simulink model "L2_Step1"  (R2021b)
settings: Solver=FixedStepDiscrete  StartTime=0.0  StopTime=inf  FixedStep=0.01  RelTol=1e-3
model workspace (MATLAB code in the model file):
  | IgnitionOff = 0;
  | IgnitionACC = 1;
  | IgnitionOnEngineOn = 2;
  | KeyAbsent = 5;
  | 
  | Active = 1;
  | Not_Active = 0;
settings Model: Creator=Ekrem Fidan  LastModifiedBy=Ekrem Fidan

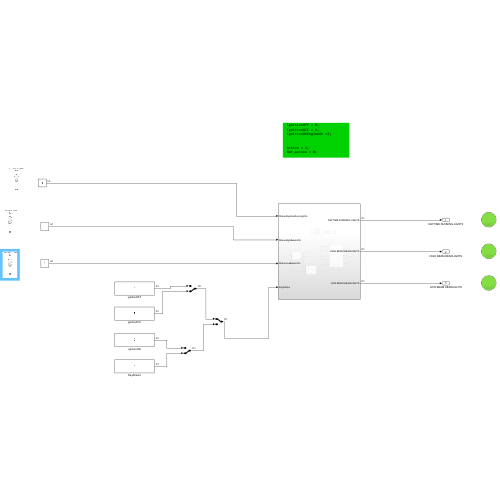
[thumbnail: Simulink's stored preview of the top-level diagram]
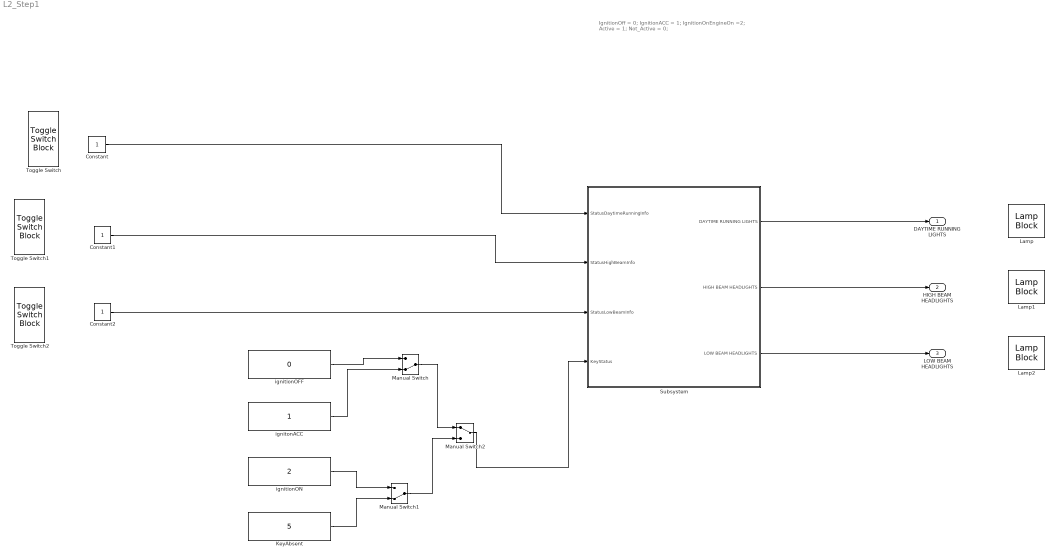
== system L2_Step1 ==
  note: IgnitionOff = 0;
      | IgnitionACC = 1;
      | IgnitionOnEngineOn =2;
      |
      | Active = 1;
      | Not_Active = 0;
  Constant : Constant
  Constant1 : Constant
  Constant2 : Constant
  KeyAbsent : Constant  Value=5  SampleTime=-1
  Lamp : LampBlock  LabelPosition=Hide
  Lamp1 : LampBlock  LabelPosition=Hide
  Lamp2 : LampBlock  LabelPosition=Hide
  Manual Switch : ManualSwitch  CurrentSetting=0
  Manual Switch1 : ManualSwitch  CurrentSetting=0
  Manual Switch2 : ManualSwitch
  Subsystem : Subsystem
  Toggle Switch : ToggleSwitchBlock
      settings: Values={{'Off', 'On'}, [0 1]}
  Toggle Switch1 : ToggleSwitchBlock
      settings: Values={{'Off', 'On'}, [0 1]}
  Toggle Switch2 : ToggleSwitchBlock
      settings: Values={{'Off', 'On'}, [0 1]}
  ignitionOFF : Constant  Value=0  SampleTime=-1
  ignitionON : Constant  Value=2  SampleTime=-1
  ignitonACC : Constant  SampleTime=-1
  DAYTIME RUNNING LIGHTS : Outport
  HIGH BEAM HEADLIGHTS : Outport  Port=2
  LOW BEAM HEADLIGHTS : Outport  Port=3
  wires:
  ignitionOFF/1 -> Manual Switch/1
  ignitonACC/1 -> Manual Switch/2
  ignitionON/1 -> Manual Switch1/1
  KeyAbsent/1 -> Manual Switch1/2
  Manual Switch/1 -> Manual Switch2/1
  Manual Switch1/1 -> Manual Switch2/2
  Constant/1 -> Subsystem/1(StatusDaytimeRunningInfo)
  Constant1/1 -> Subsystem/2(StatusHighBeamInfo)
  Constant2/1 -> Subsystem/3(StatusLowBeamInfo)
  Manual Switch2/1 -> Subsystem/4(KeyStatus)
  Subsystem/1(DAYTIME RUNNING LIGHTS) -> DAYTIME RUNNING LIGHTS/1
  Subsystem/2(HIGH BEAM HEADLIGHTS) -> HIGH BEAM HEADLIGHTS/1
  Subsystem/3(LOW BEAM HEADLIGHTS) -> LOW BEAM HEADLIGHTS/1

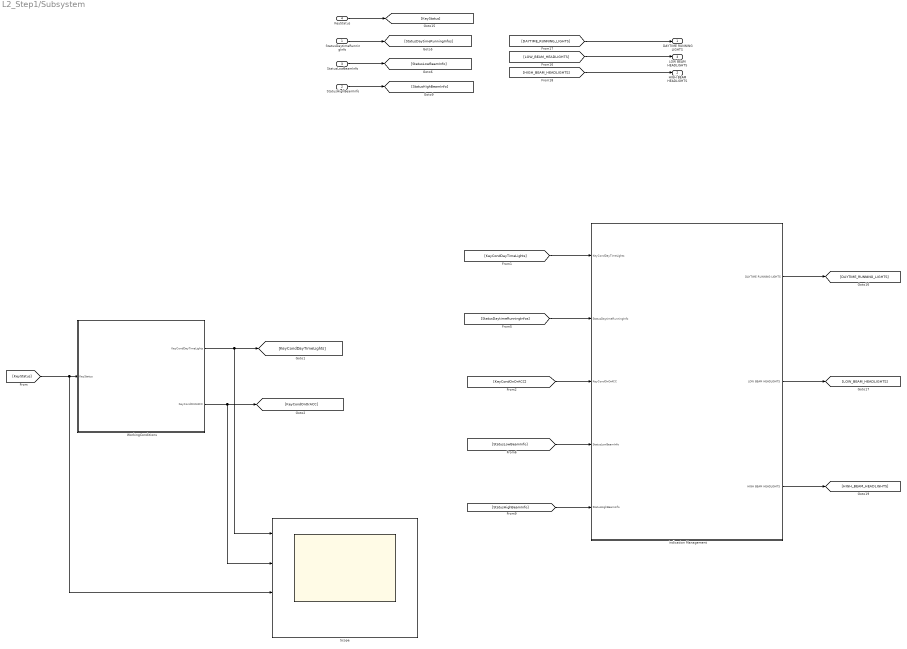
== system L2_Step1/Subsystem ==
  StatusDaytimeRunningInfo : Inport
  StatusHighBeamInfo : Inport  Port=2
  StatusLowBeamInfo : Inport  Port=3
  KeyStatus : Inport  Port=4
  Scope : Scope  NumInputPorts=4
  WorkingConditions : Subsystem
  indication Management : Subsystem
  DAYTIME RUNNING LIGHTS : Outport
  HIGH BEAM HEADLIGHTS : Outport  Port=2
  LOW BEAM HEADLIGHTS : Outport  Port=3
  wires:
  [HIGH_BEAM_HEADLIGHTS] -> HIGH BEAM HEADLIGHTS/1
  WorkingConditions/2(KeyCondOnOrACC) -> Scope/2, [KeyCondOnOrACC]
  [StatusHighBeamInfo] -> indication Management/5(StatusHighBeamInfo)
  [KeyCondOnOrACC] -> indication Management/3(KeyCondOnOrACC)
  indication Management/2(LOW BEAM HEADLIGHTS) -> [LOW_BEAM_HEADLIGHTS]
  WorkingConditions/1(KeyCondDayTimeLights) -> Scope/1, [KeyCondDayTimeLights]
  [DAYTIME_RUNNING_LIGHTS] -> DAYTIME RUNNING LIGHTS/1
  [StatusLowBeamInfo] -> indication Management/4(StatusLowBeamInfo)
  StatusDaytimeRunningInfo/1 -> [StatusDaytimeRunningInfos]
  indication Management/1(DAYTIME RUNNING LIGHTS) -> [DAYTIME_RUNNING_LIGHTS]
  [KeyCondDayTimeLights] -> indication Management/1(KeyCondDayTimeLights)
  [StatusDaytimeRunningInfos] -> indication Management/2(StatusDaytimeRunningInfo)
  StatusLowBeamInfo/1 -> [StatusLowBeamInfo]
  indication Management/3(HIGH BEAM HEADLIGHTS) -> [HIGH_BEAM_HEADLIGHTS]
  StatusHighBeamInfo/1 -> [StatusHighBeamInfo]
  [LOW_BEAM_HEADLIGHTS] -> LOW BEAM HEADLIGHTS/1
  KeyStatus/1 -> [KeyStatus]
  [KeyStatus] -> Scope/3, WorkingConditions/1(KeyStatus)

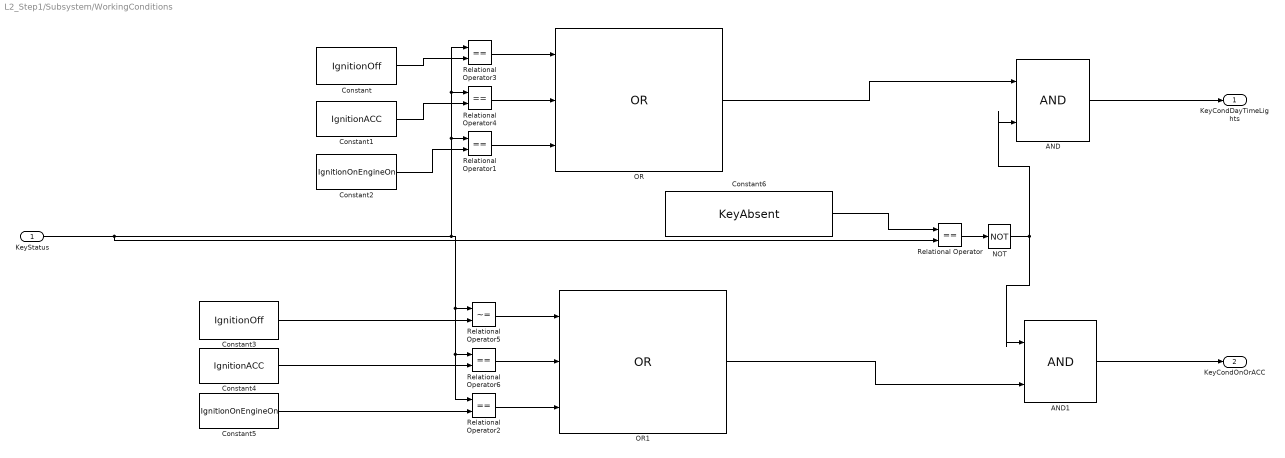
== system L2_Step1/Subsystem/WorkingConditions ==
  KeyStatus : Inport
  AND : Logic  IconShape=distinctive  AllPortsSameDT=off  OutDataTypeStr=boolean
  AND1 : Logic  IconShape=distinctive  AllPortsSameDT=off  OutDataTypeStr=boolean
  Constant : Constant  Value=IgnitionOff  SampleTime=-1
  Constant1 : Constant  Value=IgnitionACC  SampleTime=-1
  Constant2 : Constant  Value=IgnitionOnEngineOn  SampleTime=-1
  Constant3 : Constant  Value=IgnitionOff  SampleTime=-1
  Constant4 : Constant  Value=IgnitionACC  SampleTime=-1
  Constant5 : Constant  Value=IgnitionOnEngineOn  SampleTime=-1
  Constant6 : Constant  Value=KeyAbsent
  NOT : Logic  Operator=NOT  IconShape=distinctive  AllPortsSameDT=off  OutDataTypeStr=boolean
  OR : Logic  Operator=OR  Inputs=3  IconShape=distinctive  AllPortsSameDT=off  OutDataTypeStr=boolean
  OR1 : Logic  Operator=OR  Inputs=3  IconShape=distinctive  AllPortsSameDT=off  OutDataTypeStr=boolean
  Relational Operator{,1..4,6} (6 alike) : RelationalOperator  Operator===  OutDataTypeStr=boolean  RndMeth=Simplest
  Relational Operator5 : RelationalOperator  Operator=~=  OutDataTypeStr=boolean  RndMeth=Simplest
  KeyCondDayTimeLights : Outport
  KeyCondOnOrACC : Outport  Port=2
  wires:
  Constant1/1 -> Relational Operator4/2
  Relational Operator3/1 -> OR/1
  Constant/1 -> Relational Operator3/2
  Relational Operator4/1 -> OR/2
  Relational Operator1/1 -> OR/3
  Constant2/1 -> Relational Operator1/2
  Constant5/1 -> Relational Operator2/2
  Relational Operator2/1 -> OR1/3
  Relational Operator6/1 -> OR1/2
  Constant3/1 -> Relational Operator5/2
  Relational Operator5/1 -> OR1/1
  Constant4/1 -> Relational Operator6/2
  KeyStatus/1 -> Relational Operator/2, Relational Operator2/1, Relational Operator6/1, Relational Operator5/1, Relational Operator1/1, Relational Operator4/1, Relational Operator3/1
  Constant6/1 -> Relational Operator/1
  Relational Operator/1 -> NOT/1
  NOT/1 -> AND1/1, AND/2
  OR/1 -> AND/1
  OR1/1 -> AND1/2
  AND1/1 -> KeyCondOnOrACC/1
  AND/1 -> KeyCondDayTimeLights/1

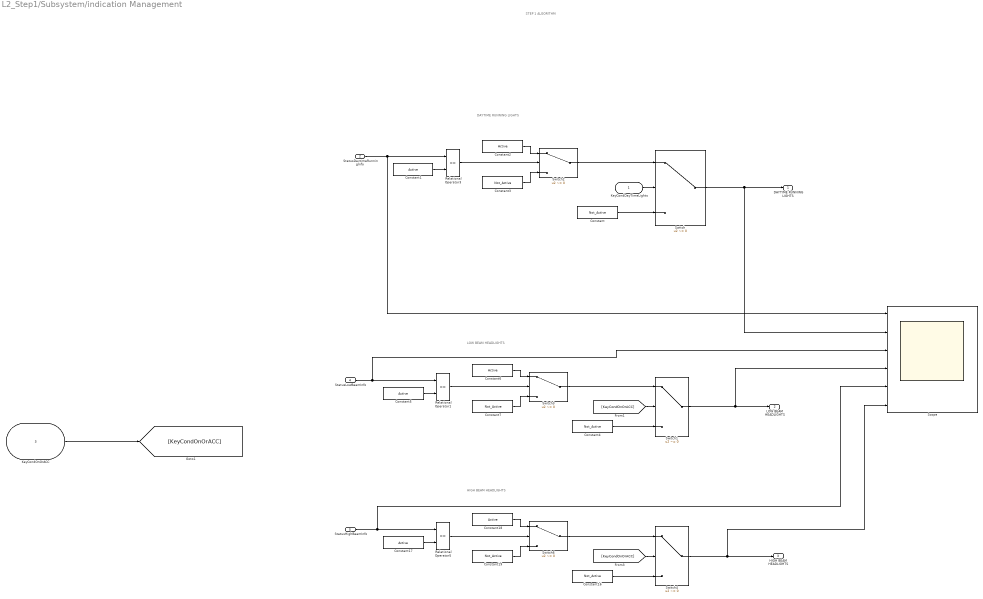
== system L2_Step1/Subsystem/indication Management ==
  note: STEP 1 ALGORITHM
  note: DAYTIME RUNNING LIGHTS
  note: LOW BEAM HEADLIGHTS
  note: HIGH BEAM HEADLIGHTS
  KeyCondDayTimeLights : Inport
  StatusDaytimeRunningInfo : Inport  Port=2
  KeyCondOnOrACC : Inport  Port=3
  StatusLowBeamInfo : Inport  Port=4
  StatusHighBeamInfo : Inport  Port=5
  Constant{,3..4,7,16,19} (6 alike) : Constant  Value=Not_Active  SampleTime=-1
  Constant{1..2,5..6,17..18} (6 alike) : Constant  Value=Active  SampleTime=-1
  Relational Operator1 : RelationalOperator  Operator===  OutDataTypeStr=boolean  RndMeth=Simplest
  Relational Operator3 : RelationalOperator  Operator===  OutDataTypeStr=boolean  RndMeth=Simplest
  Relational Operator5 : RelationalOperator  Operator===  OutDataTypeStr=boolean  RndMeth=Simplest
  Scope : Scope  NumInputPorts=6
  Switch{,1..4,6} (6 alike) : Switch  Criteria=u2 ~= 0
  DAYTIME RUNNING LIGHTS : Outport
  LOW BEAM HEADLIGHTS : Outport  Port=2
  HIGH BEAM HEADLIGHTS : Outport  Port=3
  wires:
  Constant1/1 -> Relational Operator3/2
  KeyCondDayTimeLights/1 -> Switch/2
  Switch2/1 -> Switch/1
  Constant2/1 -> Switch2/1
  Switch/1 -> Scope/2, DAYTIME RUNNING LIGHTS/1
  Constant/1 -> Switch/3
  Constant3/1 -> Switch2/3
  Relational Operator3/1 -> Switch2/2
  StatusDaytimeRunningInfo/1 -> Scope/1, Relational Operator3/1
  StatusLowBeamInfo/1 -> Scope/3, Relational Operator1/1
  Relational Operator1/1 -> Switch3/2
  Constant7/1 -> Switch3/3
  Constant4/1 -> Switch1/3
  Constant6/1 -> Switch3/1
  Switch3/1 -> Switch1/1
  [KeyCondOnOrACC] -> Switch1/2
  Constant5/1 -> Relational Operator1/2
  KeyCondOnOrACC/1 -> [KeyCondOnOrACC]
  Constant17/1 -> Relational Operator5/2
  [KeyCondOnOrACC] -> Switch4/2
  Switch6/1 -> Switch4/1
  Constant18/1 -> Switch6/1
  Constant16/1 -> Switch4/3
  Constant19/1 -> Switch6/3
  Relational Operator5/1 -> Switch6/2
  StatusHighBeamInfo/1 -> Scope/5, Relational Operator5/1
  Switch4/1 -> Scope/6, HIGH BEAM HEADLIGHTS/1
  Switch1/1 -> Scope/4, LOW BEAM HEADLIGHTS/1
